simulink model "grid_traditional"  (R2023b)
settings: Solver=ode23s  StartTime=0.0  StopTime=32  RelTol=1e-3
values from neighbouring files (symbols this model uses):
  Ts = 5e-6    (= 5e-06)    [model_parameters.m]
undefined symbols (not defined in the file or in its folder): gcbh, Grid, IBR, L, SG, sps_rtmsupport, TX
libraries: spsThreePhaseVIMeasurementLib x13, spsFourierLib x13, spsPowerPositiveSequenceLib x13, spsThreePhaseSeriesRLCLoadLib x11, spsThreePhaseSeriesRLCBranchLib x10, spsThreePhaseTransformerTwoWindingsLib x10, spsDCVoltageSourceLib x8, spsFirstOrderFilterLib x8, spsabctodq0Lib x8, spsSimplifiedSynchronousMachinepuUnitsLib x6, spsGroundLib x4, spsUniversalBridgeLib x4
(part 1 of 2)
settings Model: SimulationMode=rapid-accelerator  Creator=psernatorre  LastModifiedBy=psernatorre
settings DataIOCC: InitialState=initial_data_trad2.xFinal  LoadInitialState=on  SaveFinalState=on  SaveOperatingPoint=on
settings GRTTargetCC: RTWCAPISignals=on  RTWCAPIParams=on

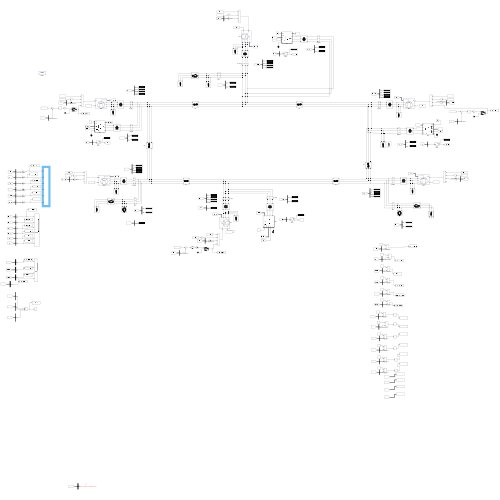
[thumbnail: Simulink's stored preview of the top-level diagram]
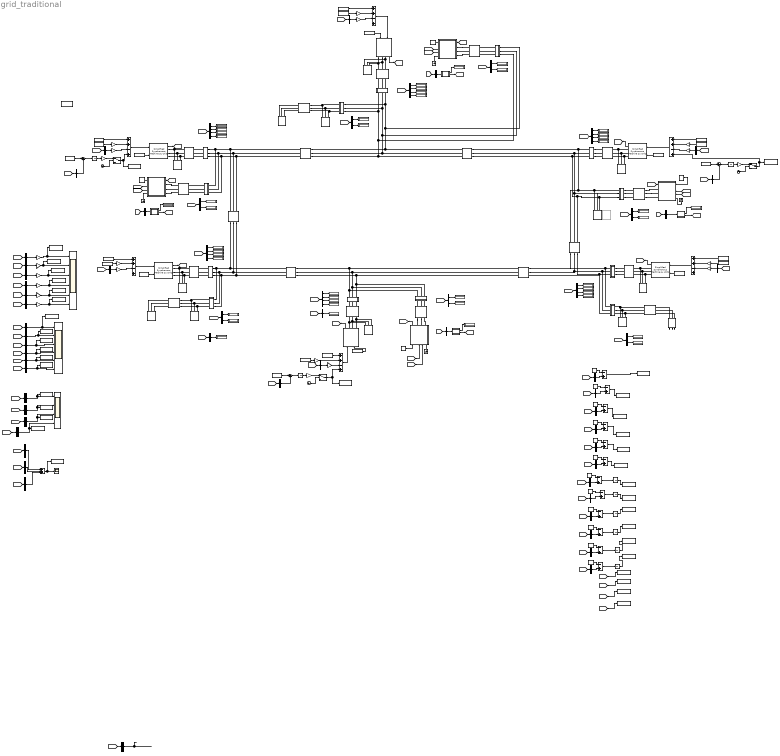
== system grid_traditional ==
  Add{,6..7,20..22} (6 alike) : Sum  Inputs=++-+
  Add1 : Sum  Inputs=+++
  Add{9,11..13,17..18,33..38} (12 alike) : Sum  Inputs=-+
  B1_IBR1 : Subsystem  mask{Sbase=Grid.Sbase, Vbase=Grid.Vbase, f=Grid.f, Ts=Ts, label=B1_IBR1, enable_power_calc=on}
      mask prompts: Sbase "Sbase (3-phase VA)"; Vbase "Vbase (L-L Vrms)"; f "Frequency (Hz)"; Ts "Sample time (s)"; label "Measure label"; enable_power_calc "Enable power calculation"
      mask init:
      | set_param([gcb '/signal'],'GotoTag', label)
      mask DialogControl DescGroupVar Prompt: Bus and measurements
      mask DialogControl Bus Prompt: Measure voltage, magnitude and phase, active power, reactive power
  B1_SG1 : Subsystem  mask{Sbase=Grid.Sbase, Vbase=Grid.Vbase, f=Grid.f, Ts=Ts, label=B1_SG1, enable_power_calc=on}
      mask prompts: Sbase "Sbase (3-phase VA)"; Vbase "Vbase (L-L Vrms)"; f "Frequency (Hz)"; Ts "Sample time (s)"; label "Measure label"; enable_power_calc "Enable power calculation"
      mask init:
      | set_param([gcb '/signal'],'GotoTag', label)
      mask DialogControl DescGroupVar Prompt: Bus and measurements
      mask DialogControl Bus Prompt: Measure voltage, magnitude and phase, active power, reactive power
  B5_L : Subsystem  mask{Sbase=Grid.Sbase, Vbase=Grid.Vbase, f=Grid.f, Ts=Ts, label=B5_L, enable_power_calc=on}
      mask prompts: Sbase "Sbase (3-phase VA)"; Vbase "Vbase (L-L Vrms)"; f "Frequency (Hz)"; Ts "Sample time (s)"; label "Measure label"; enable_power_calc "Enable power calculation"
      mask init:
      | set_param([gcb '/signal'],'GotoTag', label)
      mask DialogControl DescGroupVar Prompt: Bus and measurements
      mask DialogControl Bus Prompt: Measure voltage, magnitude and phase, active power, reactive power
  B5_SG6 : Subsystem  mask{Sbase=Grid.Sbase, Vbase=Grid.Vbase, f=Grid.f, Ts=Ts, label=B5_SG6, enable_power_calc=on}
      mask prompts: Sbase "Sbase (3-phase VA)"; Vbase "Vbase (L-L Vrms)"; f "Frequency (Hz)"; Ts "Sample time (s)"; label "Measure label"; enable_power_calc "Enable power calculation"
      mask init:
      | set_param([gcb '/signal'],'GotoTag', label)
      mask DialogControl DescGroupVar Prompt: Bus and measurements
      mask DialogControl Bus Prompt: Measure voltage, magnitude and phase, active power, reactive power
  B6_IBR3 : Subsystem  mask{Sbase=Grid.Sbase, Vbase=Grid.Vbase, f=Grid.f, Ts=Ts, label=B6_IBR3, enable_power_calc=on}
      mask prompts: Sbase "Sbase (3-phase VA)"; Vbase "Vbase (L-L Vrms)"; f "Frequency (Hz)"; Ts "Sample time (s)"; label "Measure label"; enable_power_calc "Enable power calculation"
      mask init:
      | set_param([gcb '/signal'],'GotoTag', label)
      mask DialogControl DescGroupVar Prompt: Bus and measurements
      mask DialogControl Bus Prompt: Measure voltage, magnitude and phase, active power, reactive power
  B6_SG5 : Subsystem  mask{Sbase=Grid.Sbase, Vbase=Grid.Vbase, f=Grid.f, Ts=Ts, label=B6_SG5, enable_power_calc=on}
      mask prompts: Sbase "Sbase (3-phase VA)"; Vbase "Vbase (L-L Vrms)"; f "Frequency (Hz)"; Ts "Sample time (s)"; label "Measure label"; enable_power_calc "Enable power calculation"
      mask init:
      | set_param([gcb '/signal'],'GotoTag', label)
      mask DialogControl DescGroupVar Prompt: Bus and measurements
      mask DialogControl Bus Prompt: Measure voltage, magnitude and phase, active power, reactive power
  B7_IBR4 : Subsystem  mask{Sbase=Grid.Sbase, Vbase=Grid.Vbase, f=Grid.f, Ts=Ts, label=B7_IBR4, enable_power_calc=on}
      mask prompts: Sbase "Sbase (3-phase VA)"; Vbase "Vbase (L-L Vrms)"; f "Frequency (Hz)"; Ts "Sample time (s)"; label "Measure label"; enable_power_calc "Enable power calculation"
      mask init:
      | set_param([gcb '/signal'],'GotoTag', label)
      mask DialogControl DescGroupVar Prompt: Bus and measurements
      mask DialogControl Bus Prompt: Measure voltage, magnitude and phase, active power, reactive power
  B7_L : Subsystem  mask{Sbase=Grid.Sbase, Vbase=Grid.Vbase, f=Grid.f, Ts=Ts, label=B7_L, enable_power_calc=on}
      mask prompts: Sbase "Sbase (3-phase VA)"; Vbase "Vbase (L-L Vrms)"; f "Frequency (Hz)"; Ts "Sample time (s)"; label "Measure label"; enable_power_calc "Enable power calculation"
      mask init:
      | set_param([gcb '/signal'],'GotoTag', label)
      mask DialogControl DescGroupVar Prompt: Bus and measurements
      mask DialogControl Bus Prompt: Measure voltage, magnitude and phase, active power, reactive power
  B7_SG4 : Subsystem  mask{Sbase=Grid.Sbase, Vbase=Grid.Vbase, f=Grid.f, Ts=Ts, label=B7_SG4, enable_power_calc=on}
      mask prompts: Sbase "Sbase (3-phase VA)"; Vbase "Vbase (L-L Vrms)"; f "Frequency (Hz)"; Ts "Sample time (s)"; label "Measure label"; enable_power_calc "Enable power calculation"
      mask init:
      | set_param([gcb '/signal'],'GotoTag', label)
      mask DialogControl DescGroupVar Prompt: Bus and measurements
      mask DialogControl Bus Prompt: Measure voltage, magnitude and phase, active power, reactive power
  B8_IBR2 : Subsystem  mask{Sbase=Grid.Sbase, Vbase=Grid.Vbase, f=Grid.f, Ts=Ts, label=B8_IBR2, enable_power_calc=on}
      mask prompts: Sbase "Sbase (3-phase VA)"; Vbase "Vbase (L-L Vrms)"; f "Frequency (Hz)"; Ts "Sample time (s)"; label "Measure label"; enable_power_calc "Enable power calculation"
      mask init:
      | set_param([gcb '/signal'],'GotoTag', label)
      mask DialogControl DescGroupVar Prompt: Bus and measurements
      mask DialogControl Bus Prompt: Measure voltage, magnitude and phase, active power, reactive power
  B8_SG3 : Subsystem  mask{Sbase=Grid.Sbase, Vbase=Grid.Vbase, f=Grid.f, Ts=Ts, label=B8_SG3, enable_power_calc=on}
      mask prompts: Sbase "Sbase (3-phase VA)"; Vbase "Vbase (L-L Vrms)"; f "Frequency (Hz)"; Ts "Sample time (s)"; label "Measure label"; enable_power_calc "Enable power calculation"
      mask init:
      | set_param([gcb '/signal'],'GotoTag', label)
      mask DialogControl DescGroupVar Prompt: Bus and measurements
      mask DialogControl Bus Prompt: Measure voltage, magnitude and phase, active power, reactive power
  B9_L : Subsystem  mask{Sbase=Grid.Sbase, Vbase=Grid.Vbase, f=Grid.f, Ts=Ts, label=B9_L, enable_power_calc=on}
      mask prompts: Sbase "Sbase (3-phase VA)"; Vbase "Vbase (L-L Vrms)"; f "Frequency (Hz)"; Ts "Sample time (s)"; label "Measure label"; enable_power_calc "Enable power calculation"
      mask init:
      | set_param([gcb '/signal'],'GotoTag', label)
      mask DialogControl DescGroupVar Prompt: Bus and measurements
      mask DialogControl Bus Prompt: Measure voltage, magnitude and phase, active power, reactive power
  B9_SG2 : Subsystem  mask{Sbase=Grid.Sbase, Vbase=Grid.Vbase, f=Grid.f, Ts=Ts, label=B9_SG2, enable_power_calc=on}
      mask prompts: Sbase "Sbase (3-phase VA)"; Vbase "Vbase (L-L Vrms)"; f "Frequency (Hz)"; Ts "Sample time (s)"; label "Measure label"; enable_power_calc "Enable power calculation"
      mask init:
      | set_param([gcb '/signal'],'GotoTag', label)
      mask DialogControl DescGroupVar Prompt: Bus and measurements
      mask DialogControl Bus Prompt: Measure voltage, magnitude and phase, active power, reactive power
  Bus Selector{1,29,31,33,91..92} (6 alike) : BusSelector  OutputSignals=P,Q,Vmag,Vphase
  Bus Selector{8,10..11,19,32,42..48,55,58} (14 alike) : BusSelector  OutputSignals=P
  Bus Selector{3..7,9,12..13,16..18,20..22,24..25,28,30,34,37,39..41,49..54} (29 alike) : BusSelector  OutputSignals=Rotor speed wm (pu)
  Bus Selector{14..15,35,56} (4 alike) : BusSelector  OutputSignals=V
  Bus Selector{2,23,26..27,36,38,57} (7 alike) : BusSelector  OutputSignals=P,Q
  Clock : Clock
  Clock1 : Clock
  Clock2 : Clock
  Constant{,17,20,23..24,28} (6 alike) : Constant  Value=1.02
  Constant1 : Constant  Value=0.54
  Constant{5..14,16,18..19,22,27,36..41} (21 alike) : Constant
  Constant15 : Constant  Value=0.52
  Constant2 : Constant  Value=0.35
  Constant21 : Constant  Value=0.10
  Constant25 : Constant  Value=0.80
  Constant26 : Constant  Value=0.70
  Constant29 : Constant  Value=0.15
  Constant3 : Constant  Value=0.35
  Constant30 : Constant  Value=0.30
  Constant4 : Constant  Value=0.35
  Display{1..44} (44 alike) : Display
      settings: Format=bank
  Gain{1,10..11,26..28} (6 alike) : Gain  Gain=Grid.f
  Gain12 : Gain  Gain=1/SG(4).Rp
  Gain17 : Gain  Gain=1/SG(2).Rp
  Gain18 : Gain  Gain=1/SG(2).Rp
  Gain19 : Gain  Gain=1/SG(3).Rp
  Gain2 : Gain  Gain=1/SG(1).Rp
  Gain20 : Gain  Gain=1/SG(3).Rp
  Gain21 : Gain  Gain=1/SG(4).Rp
  Gain22 : Gain  Gain=1/SG(5).Rp
  Gain23 : Gain  Gain=1/SG(5).Rp
  Gain24 : Gain  Gain=1/SG(6).Rp
  Gain25 : Gain  Gain=1/SG(6).Rp
  Gain3 : Gain  Gain=1/SG(1).Rp
  Gain4 : Gain  Gain=40
  Gain5 : Gain  Gain=40
  Gain6 : Gain  Gain=40
  Ground{1..4} (4 alike) : spsGroundLib/Ground  LConnTagsString=a
  IBR1 : Subsystem  mask{S=Grid.Sbase, V=IBR(1).Vbase, Vdc=IBR(1).Vdc, Rf=IBR(1).Rf, Lf=IBR(1).Lf, Rc=IBR(1).Rc, Lc=IBR(1).Lc, Kp=IBR(1).Kp, Ki=IBR(1).Ki, f=Grid.f, Tf=IBR(1).Tf, Ts=Ts, enable_state_estimation=off, A_est=0, B_est=0, C_est=0, D_est=0}
      mask prompts: S "Pnom (VA)"; V "Vnom (Line Vrms)"; Vdc "Vdc (V)"; Rf "Rf (p.u.)"; Lf "Lf (p.u.)"; Rc "Rc (p.u.)"; Lc "Lc (p.u.)"; f "Frequency (Hz)"; Tf "Tf (feed-forward)"; Ts "Sample time (s)"; enable_state_estimation "Enable state estimation"
      mask DialogControl DescGroupVar Prompt: PLL-based grid-following IBR with LC filter
      mask DialogControl DescTextVar Prompt: Implements a grid-following inverter with LC filter with PI controllers in dq0-synchronous frames. It considers feed-forward compensation with first-order low-pass filter. Rf and Lf are impendances of the internal filter, and Rc and Lc are the impendances including a step-up transformer if there exists.
      mask Display: image('GFL_LC.png');
  IBR2 : Subsystem  mask{S=Grid.Sbase, V=IBR(2).Vbase, Vdc=IBR(2).Vdc, Rf=IBR(2).Rf, Lf=IBR(2).Lf, Rc=IBR(2).Rc, Lc=IBR(2).Lc, Kp=IBR(2).Kp, Ki=IBR(2).Ki, f=Grid.f, Tf=IBR(2).Tf, Ts=Ts, enable_state_estimation=off, A_est=0, B_est=0, C_est=0, D_est=0}
      mask prompts: S "Pnom (VA)"; V "Vnom (Line Vrms)"; Vdc "Vdc (V)"; Rf "Rf (p.u.)"; Lf "Lf (p.u.)"; Rc "Rc (p.u.)"; Lc "Lc (p.u.)"; f "Frequency (Hz)"; Tf "Tf (feed-forward)"; Ts "Sample time (s)"; enable_state_estimation "Enable state estimation"
      mask DialogControl DescGroupVar Prompt: PLL-based grid-following IBR with LC filter
      mask DialogControl DescTextVar Prompt: Implements a grid-following inverter with LC filter with PI controllers in dq0-synchronous frames. It considers feed-forward compensation with first-order low-pass filter. Rf and Lf are impendances of the internal filter, and Rc and Lc are the impendances including a step-up transformer if there exists.
      mask Display: image('GFL_LC.png');
  IBR3 : Subsystem  mask{S=Grid.Sbase, V=IBR(3).Vbase, Vdc=IBR(3).Vdc, Rf=IBR(3).Rf, Lf=IBR(3).Lf, Rc=IBR(3).Rc, Lc=IBR(3).Lc, Kp=IBR(3).Kp, Ki=IBR(3).Ki, f=Grid.f, Tf=IBR(3).Tf, Ts=Ts, enable_state_estimation=off, A_est=0, B_est=0, C_est=0, D_est=0}
      mask prompts: S "Pnom (VA)"; V "Vnom (Line Vrms)"; Vdc "Vdc (V)"; Rf "Rf (p.u.)"; Lf "Lf (p.u.)"; Rc "Rc (p.u.)"; Lc "Lc (p.u.)"; f "Frequency (Hz)"; Tf "Tf (feed-forward)"; Ts "Sample time (s)"; enable_state_estimation "Enable state estimation"
      mask DialogControl DescGroupVar Prompt: PLL-based grid-following IBR with LC filter
      mask DialogControl DescTextVar Prompt: Implements a grid-following inverter with LC filter with PI controllers in dq0-synchronous frames. It considers feed-forward compensation with first-order low-pass filter. Rf and Lf are impendances of the internal filter, and Rc and Lc are the impendances including a step-up transformer if there exists.
      mask Display: image('GFL_LC.png');
  IBR4 : Subsystem  mask{S=Grid.Sbase, V=IBR(2).Vbase, Vdc=IBR(2).Vdc, Rf=IBR(2).Rf, Lf=IBR(2).Lf, Rc=IBR(2).Rc, Lc=IBR(2).Lc, Kp=IBR(2).Kp, Ki=IBR(2).Ki, f=Grid.f, Tf=IBR(2).Tf, Ts=Ts, enable_state_estimation=off, A_est=0, B_est=0, C_est=0, D_est=0}
      mask prompts: S "Pnom (VA)"; V "Vnom (Line Vrms)"; Vdc "Vdc (V)"; Rf "Rf (p.u.)"; Lf "Lf (p.u.)"; Rc "Rc (p.u.)"; Lc "Lc (p.u.)"; f "Frequency (Hz)"; Tf "Tf (feed-forward)"; Ts "Sample time (s)"; enable_state_estimation "Enable state estimation"
      mask DialogControl DescGroupVar Prompt: PLL-based grid-following IBR with LC filter
      mask DialogControl DescTextVar Prompt: Implements a grid-following inverter with LC filter with PI controllers in dq0-synchronous frames. It considers feed-forward compensation with first-order low-pass filter. Rf and Lf are impendances of the internal filter, and Rc and Lc are the impendances including a step-up transformer if there exists.
      mask Display: image('GFL_LC.png');
  Integrator{,1..5,12..14} (9 alike) : Integrator
  PLL (3ph) : Subsystem  AncestorBlock=|  DialogController=POWERSYS.PowerSysDialog  LoadFcn=sps_rtmsupport('LoadFcn', gcbh);  StartFcn=sps_rtmsupport('StartFcn', gcbh);  StopFcn=sps_rtmsupport('StopFcn', gcbh);  mask(PLL (3ph)){Fmin=45, Par_Init=[0, 60], ParK=[180, 3200, 1], TcD=1e-4, MaxRateChangeFreq=12, FilterCutOffFreq=25, Ts=Ts, AGC=on}
      | sps_lib/Control/PLL
      | (3ph)
      mask prompts: Fmin "Minimum frequency (Hz):"; Par_Init "Initial inputs [ Phase (degrees), Frequency (Hz) ]:"; ParK "Regulator gains [ Kp, Ki, Kd ]:"; TcD "Time constant for derivative action (s):"; MaxRateChangeFreq "Maximum rate of change of frequency (Hz/s):"; FilterCutOffFreq "Filter cut-off frequency for frequency measurement (Hz):"; Ts "Sample time:"; AGC "Enable automatic gain control"
      mask help:
      | This Phase Locked Loop (PLL) system can be used  to synchronize on a set of variable frequency, three-phase sinusoidal signals. If the Automatic Gain Control is enabled, the input (phase error) of the PLL regulator is scaled according to the input signals magnitude.
      |
      | For optimal performance, set regulator gains [ Kp Ki  Kd ] = [ 180  3200  1 ] and check the Enable Automatic Gain Control parameter.
      |
      | Input : Vector containing the normalized three-phase signals [Va Vb Vc]
      | Output 1:  Measured frequency (Hz) = w/(2pi)
      | Output 2:  Ramp w.t varying between  0 and 2*pi, synchronized on zero crossings of the fundamental (positive-sequence) of phase A.
      mask init:
      | block=gcb;
      | [WantBlockChoice,Ts,sps] = powericon('PLL3phInit',block,Fmin,Par_Init,ParK,TcD, MaxRateChangeFreq, FilterCutOffFreq, AGC,Ts);
      | powericon('SetInternalModels','set',block,WantBlockChoice);
      settings: CopyFcn=sps_rtmsupport('CopyFcn', gcbh);  DeleteFcn=sps_rtmsupport('DeleteFcn', gcbh);  UndoDeleteFcn=sps_rtmsupport('UndoDeleteFcn', gcbh);  ModelCloseFcn=sps_rtmsupport('ModelCloseFcn', gcbh);  PreSaveFcn=sps_rtmsupport('PreSaveFcn', gcbh);  PostSaveFcn=sps_rtmsupport('PostSaveFcn', gcbh);  NameChangeFcn=sps_rtmsupport('NameChangeFcn', gcbh);  PreCopyFcn=sps_rtmsupport('PreCopyFcn', gcbh);  OpenFcn=sps_rtmsupport('OpenFcn', gcbh, [8]);  CloseFcn=sps_rtmsupport('CloseFcn', gcbh);  PreDeleteFcn=sps_rtmsupport('PreDeleteFcn', gcbh);
      settings: LibrarySourceBlock=|
      | sps_lib/Control/PLL
      | (3ph)
      mask Help: helpview(psbhelp);
  PLL (3ph)1 : Subsystem  AncestorBlock=|  DialogController=POWERSYS.PowerSysDialog  LoadFcn=sps_rtmsupport('LoadFcn', gcbh);  StartFcn=sps_rtmsupport('StartFcn', gcbh);  StopFcn=sps_rtmsupport('StopFcn', gcbh);  mask(PLL (3ph)){Fmin=45, Par_Init=[0, 60], ParK=[180, 3200, 1], TcD=1e-4, MaxRateChangeFreq=12, FilterCutOffFreq=25, Ts=Ts, AGC=on}
      | sps_lib/Control/PLL
      | (3ph)
      mask prompts: Fmin "Minimum frequency (Hz):"; Par_Init "Initial inputs [ Phase (degrees), Frequency (Hz) ]:"; ParK "Regulator gains [ Kp, Ki, Kd ]:"; TcD "Time constant for derivative action (s):"; MaxRateChangeFreq "Maximum rate of change of frequency (Hz/s):"; FilterCutOffFreq "Filter cut-off frequency for frequency measurement (Hz):"; Ts "Sample time:"; AGC "Enable automatic gain control"
      mask help:
      | This Phase Locked Loop (PLL) system can be used  to synchronize on a set of variable frequency, three-phase sinusoidal signals. If the Automatic Gain Control is enabled, the input (phase error) of the PLL regulator is scaled according to the input signals magnitude.
      |
      | For optimal performance, set regulator gains [ Kp Ki  Kd ] = [ 180  3200  1 ] and check the Enable Automatic Gain Control parameter.
      |
      | Input : Vector containing the normalized three-phase signals [Va Vb Vc]
      | Output 1:  Measured frequency (Hz) = w/(2pi)
      | Output 2:  Ramp w.t varying between  0 and 2*pi, synchronized on zero crossings of the fundamental (positive-sequence) of phase A.
      mask init:
      | block=gcb;
      | [WantBlockChoice,Ts,sps] = powericon('PLL3phInit',block,Fmin,Par_Init,ParK,TcD, MaxRateChangeFreq, FilterCutOffFreq, AGC,Ts);
      | powericon('SetInternalModels','set',block,WantBlockChoice);
      settings: CopyFcn=sps_rtmsupport('CopyFcn', gcbh);  DeleteFcn=sps_rtmsupport('DeleteFcn', gcbh);  UndoDeleteFcn=sps_rtmsupport('UndoDeleteFcn', gcbh);  ModelCloseFcn=sps_rtmsupport('ModelCloseFcn', gcbh);  PreSaveFcn=sps_rtmsupport('PreSaveFcn', gcbh);  PostSaveFcn=sps_rtmsupport('PostSaveFcn', gcbh);  NameChangeFcn=sps_rtmsupport('NameChangeFcn', gcbh);  PreCopyFcn=sps_rtmsupport('PreCopyFcn', gcbh);  OpenFcn=sps_rtmsupport('OpenFcn', gcbh, [8]);  CloseFcn=sps_rtmsupport('CloseFcn', gcbh);  PreDeleteFcn=sps_rtmsupport('PreDeleteFcn', gcbh);
      settings: LibrarySourceBlock=|
      | sps_lib/Control/PLL
      | (3ph)
      mask Help: helpview(psbhelp);
  PLL (3ph)2 : Subsystem  AncestorBlock=|  DialogController=POWERSYS.PowerSysDialog  LoadFcn=sps_rtmsupport('LoadFcn', gcbh);  StartFcn=sps_rtmsupport('StartFcn', gcbh);  StopFcn=sps_rtmsupport('StopFcn', gcbh);  mask(PLL (3ph)){Fmin=45, Par_Init=[0, 60], ParK=[180, 3200, 1], TcD=1e-4, MaxRateChangeFreq=12, FilterCutOffFreq=25, Ts=Ts, AGC=on}
      | sps_lib/Control/PLL
      | (3ph)
      mask prompts: Fmin "Minimum frequency (Hz):"; Par_Init "Initial inputs [ Phase (degrees), Frequency (Hz) ]:"; ParK "Regulator gains [ Kp, Ki, Kd ]:"; TcD "Time constant for derivative action (s):"; MaxRateChangeFreq "Maximum rate of change of frequency (Hz/s):"; FilterCutOffFreq "Filter cut-off frequency for frequency measurement (Hz):"; Ts "Sample time:"; AGC "Enable automatic gain control"
      mask help:
      | This Phase Locked Loop (PLL) system can be used  to synchronize on a set of variable frequency, three-phase sinusoidal signals. If the Automatic Gain Control is enabled, the input (phase error) of the PLL regulator is scaled according to the input signals magnitude.
      |
      | For optimal performance, set regulator gains [ Kp Ki  Kd ] = [ 180  3200  1 ] and check the Enable Automatic Gain Control parameter.
      |
      | Input : Vector containing the normalized three-phase signals [Va Vb Vc]
      | Output 1:  Measured frequency (Hz) = w/(2pi)
      | Output 2:  Ramp w.t varying between  0 and 2*pi, synchronized on zero crossings of the fundamental (positive-sequence) of phase A.
      mask init:
      | block=gcb;
      | [WantBlockChoice,Ts,sps] = powericon('PLL3phInit',block,Fmin,Par_Init,ParK,TcD, MaxRateChangeFreq, FilterCutOffFreq, AGC,Ts);
      | powericon('SetInternalModels','set',block,WantBlockChoice);
      settings: CopyFcn=sps_rtmsupport('CopyFcn', gcbh);  DeleteFcn=sps_rtmsupport('DeleteFcn', gcbh);  UndoDeleteFcn=sps_rtmsupport('UndoDeleteFcn', gcbh);  ModelCloseFcn=sps_rtmsupport('ModelCloseFcn', gcbh);  PreSaveFcn=sps_rtmsupport('PreSaveFcn', gcbh);  PostSaveFcn=sps_rtmsupport('PostSaveFcn', gcbh);  NameChangeFcn=sps_rtmsupport('NameChangeFcn', gcbh);  PreCopyFcn=sps_rtmsupport('PreCopyFcn', gcbh);  OpenFcn=sps_rtmsupport('OpenFcn', gcbh, [8]);  CloseFcn=sps_rtmsupport('CloseFcn', gcbh);  PreDeleteFcn=sps_rtmsupport('PreDeleteFcn', gcbh);
      settings: LibrarySourceBlock=|
      | sps_lib/Control/PLL
      | (3ph)
      mask Help: helpview(psbhelp);
  PLL (3ph)3 : Subsystem  AncestorBlock=|  DialogController=POWERSYS.PowerSysDialog  LoadFcn=sps_rtmsupport('LoadFcn', gcbh);  StartFcn=sps_rtmsupport('StartFcn', gcbh);  StopFcn=sps_rtmsupport('StopFcn', gcbh);  mask(PLL (3ph)){Fmin=45, Par_Init=[0, 60], ParK=[180, 3200, 1], TcD=1e-4, MaxRateChangeFreq=12, FilterCutOffFreq=25, Ts=Ts, AGC=on}
      | sps_lib/Control/PLL
      | (3ph)
      mask prompts: Fmin "Minimum frequency (Hz):"; Par_Init "Initial inputs [ Phase (degrees), Frequency (Hz) ]:"; ParK "Regulator gains [ Kp, Ki, Kd ]:"; TcD "Time constant for derivative action (s):"; MaxRateChangeFreq "Maximum rate of change of frequency (Hz/s):"; FilterCutOffFreq "Filter cut-off frequency for frequency measurement (Hz):"; Ts "Sample time:"; AGC "Enable automatic gain control"
      mask help:
      | This Phase Locked Loop (PLL) system can be used  to synchronize on a set of variable frequency, three-phase sinusoidal signals. If the Automatic Gain Control is enabled, the input (phase error) of the PLL regulator is scaled according to the input signals magnitude.
      |
      | For optimal performance, set regulator gains [ Kp Ki  Kd ] = [ 180  3200  1 ] and check the Enable Automatic Gain Control parameter.
      |
      | Input : Vector containing the normalized three-phase signals [Va Vb Vc]
      | Output 1:  Measured frequency (Hz) = w/(2pi)
      | Output 2:  Ramp w.t varying between  0 and 2*pi, synchronized on zero crossings of the fundamental (positive-sequence) of phase A.
      mask init:
      | block=gcb;
      | [WantBlockChoice,Ts,sps] = powericon('PLL3phInit',block,Fmin,Par_Init,ParK,TcD, MaxRateChangeFreq, FilterCutOffFreq, AGC,Ts);
      | powericon('SetInternalModels','set',block,WantBlockChoice);
      settings: CopyFcn=sps_rtmsupport('CopyFcn', gcbh);  DeleteFcn=sps_rtmsupport('DeleteFcn', gcbh);  UndoDeleteFcn=sps_rtmsupport('UndoDeleteFcn', gcbh);  ModelCloseFcn=sps_rtmsupport('ModelCloseFcn', gcbh);  PreSaveFcn=sps_rtmsupport('PreSaveFcn', gcbh);  PostSaveFcn=sps_rtmsupport('PostSaveFcn', gcbh);  NameChangeFcn=sps_rtmsupport('NameChangeFcn', gcbh);  PreCopyFcn=sps_rtmsupport('PreCopyFcn', gcbh);  OpenFcn=sps_rtmsupport('OpenFcn', gcbh, [8]);  CloseFcn=sps_rtmsupport('CloseFcn', gcbh);  PreDeleteFcn=sps_rtmsupport('PreDeleteFcn', gcbh);
      settings: LibrarySourceBlock=|
      | sps_lib/Control/PLL
      | (3ph)
      mask Help: helpview(psbhelp);
  SG1 : spsSimplifiedSynchronousMachinepuUnitsLib/Simplified Synchronous Machine pu Units  ConnectionType=3-wire Y  MechanicalLoad=Mechanical power Pm  MeasurementBus=off  NominalParameters=[SG(1).Sbase SG(1).Vbase Grid.f]  Mechanical=[SG(1).H SG(1).KD 20]  InternalRL="[0.02  0.3]"  InitialConditions=[0 6.93594 0.40802 0.40802 0.40802 0.604989 -119.395 120.605]  IterativeDiscreteModel=Trapezoidal non iterative  TsBlock=-1  TsPowergui=0  LoadFlowParameters=[1,0,0,0,0]  Units=0  BusType=swing  Pref=20000000  Qref=0  Qmin=-Inf  Qmax=Inf  PLF=0  QLF=0
      settings: LibrarySourceBlock=|
      | sps_lib/Electrical Machines/Simplified Synchronous
      | Machine pu Units
  SG2 : spsSimplifiedSynchronousMachinepuUnitsLib/Simplified Synchronous Machine pu Units  ConnectionType=3-wire Y  MechanicalLoad=Mechanical power Pm  MeasurementBus=off  NominalParameters=[SG(2).Sbase SG(2).Vbase Grid.f]  Mechanical=[SG(2).H SG(2).KD 20]  InternalRL="[0.02  0.3]"  InitialConditions=[0 1.16591 0.202284 0.202284 0.202284 -10.8065 -130.807 109.193]  IterativeDiscreteModel=Trapezoidal non iterative  TsBlock=-1  TsPowergui=0  LoadFlowParameters=[1,0,0,0,0]  Units=0  BusType=PV  Pref=20000000  Qref=0  Qmin=-Inf  Qmax=Inf  PLF=0  QLF=0
      settings: LibrarySourceBlock=|
      | sps_lib/Electrical Machines/Simplified Synchronous
      | Machine pu Units
  SG3 : spsSimplifiedSynchronousMachinepuUnitsLib/Simplified Synchronous Machine pu Units  ConnectionType=3-wire Y  MechanicalLoad=Mechanical power Pm  MeasurementBus=off  NominalParameters=[SG(3).Sbase SG(3).Vbase Grid.f]  Mechanical=[SG(3).H SG(3).KD 20]  InternalRL="[0.02  0.3]"  InitialConditions=[0 2.15966 0.200038 0.200038 0.200038 -0.157653 -120.158 119.842]  IterativeDiscreteModel=Trapezoidal non iterative  TsBlock=-1  TsPowergui=0  LoadFlowParameters=[1,0,0,0,0]  Units=0  BusType=PV  Pref=20000000  Qref=0  Qmin=-Inf  Qmax=Inf  PLF=0  QLF=0
      settings: LibrarySourceBlock=|
      | sps_lib/Electrical Machines/Simplified Synchronous
      | Machine pu Units
  SG4 : spsSimplifiedSynchronousMachinepuUnitsLib/Simplified Synchronous Machine pu Units  ConnectionType=3-wire Y  MechanicalLoad=Mechanical power Pm  MeasurementBus=off  NominalParameters=[SG(4).Sbase SG(4).Vbase Grid.f]  Mechanical=[SG(4).H SG(4).KD 20]  InternalRL="[0.02  0.3]"  InitialConditions=[0 -3.45004 0.102056 0.102056 0.102056 -16.653 -136.653 103.347]  IterativeDiscreteModel=Trapezoidal non iterative  TsBlock=-1  TsPowergui=0  LoadFlowParameters=[1,0,0,0,0]  Units=0  BusType=PV  Pref=10000000  Qref=0  Qmin=-Inf  Qmax=Inf  PLF=0  QLF=0
      settings: LibrarySourceBlock=|
      | sps_lib/Electrical Machines/Simplified Synchronous
      | Machine pu Units
  SG5 : spsSimplifiedSynchronousMachinepuUnitsLib/Simplified Synchronous Machine pu Units  ConnectionType=3-wire Y  MechanicalLoad=Mechanical power Pm  MeasurementBus=off  NominalParameters=[SG(5).Sbase SG(5).Vbase Grid.f]  Mechanical=[SG(5).H SG(5).KD 20]  InternalRL="[0.02  0.3]"  InitialConditions=[0 -3.45004 0.102056 0.102056 0.102056 -16.653 -136.653 103.347]  IterativeDiscreteModel=Trapezoidal non iterative  TsBlock=-1  TsPowergui=0  LoadFlowParameters=[1,0,0,0,0]  Units=0  BusType=PV  Pref=10000000  Qref=0  Qmin=-Inf  Qmax=Inf  PLF=0  QLF=0
      settings: LibrarySourceBlock=|
      | sps_lib/Electrical Machines/Simplified Synchronous
      | Machine pu Units
  SG6 : spsSimplifiedSynchronousMachinepuUnitsLib/Simplified Synchronous Machine pu Units  ConnectionType=3-wire Y  MechanicalLoad=Mechanical power Pm  MeasurementBus=off  NominalParameters=[SG(6).Sbase SG(6).Vbase Grid.f]  Mechanical=[SG(6).H SG(6).KD 20]  InternalRL="[0.02  0.3]"  InitialConditions=[0 -3.45004 0.102056 0.102056 0.102056 -16.653 -136.653 103.347]  IterativeDiscreteModel=Trapezoidal non iterative  TsBlock=-1  TsPowergui=0  LoadFlowParameters=[1,0,0,0,0]  Units=0  BusType=PV  Pref=10000000  Qref=0  Qmin=-Inf  Qmax=Inf  PLF=0  QLF=0
      settings: LibrarySourceBlock=|
      | sps_lib/Electrical Machines/Simplified Synchronous
      | Machine pu Units
  Scope : Scope  NumInputPorts=6
  Scope1 : Scope  NumInputPorts=6
  Scope2 : Scope  NumInputPorts=4
  Scope3 : Scope
  Sum : Sum  Inputs=|+-
  Sum1 : Sum  Inputs=|+-
  Sum2 : Sum  Inputs=|+-
  Switch : Switch  Threshold=3  SaturateOnIntegerOverflow=off  InputSameDT=off
  Switch1 : Switch  Threshold=3  SaturateOnIntegerOverflow=off  InputSameDT=off
  Switch2 : Switch  Threshold=3  SaturateOnIntegerOverflow=off  InputSameDT=off
  TX1 : spsThreePhaseSeriesRLCBranchLib/Three-Phase Series RLC Branch  LConnTagsString=A|B|C  RConnTagsString=A|B|C  BranchType=RL  Resistance=TX(1).R_ohm  Inductance=TX(1).L_H  Capacitance=1e-6  Measurements=None
  TX2 : spsThreePhaseSeriesRLCBranchLib/Three-Phase Series RLC Branch  LConnTagsString=A|B|C  RConnTagsString=A|B|C  BranchType=RL  Resistance=TX(2).R_ohm  Inductance=TX(2).L_H  Capacitance=1e-6  Measurements=None
  TX3 : spsThreePhaseSeriesRLCBranchLib/Three-Phase Series RLC Branch  LConnTagsString=A|B|C  RConnTagsString=A|B|C  BranchType=RL  Resistance=TX(3).R_ohm  Inductance=TX(3).L_H  Capacitance=1e-6  Measurements=None
  TX4 : spsThreePhaseSeriesRLCBranchLib/Three-Phase Series RLC Branch  LConnTagsString=A|B|C  RConnTagsString=A|B|C  BranchType=RL  Resistance=TX(4).R_ohm  Inductance=TX(4).L_H  Capacitance=1e-6  Measurements=None
  TX5 : spsThreePhaseSeriesRLCBranchLib/Three-Phase Series RLC Branch  LConnTagsString=A|B|C  RConnTagsString=A|B|C  BranchType=RL  Resistance=TX(5).R_ohm  Inductance=TX(5).L_H  Capacitance=1e-6  Measurements=None
  TX6 : spsThreePhaseSeriesRLCBranchLib/Three-Phase Series RLC Branch  LConnTagsString=A|B|C  RConnTagsString=A|B|C  BranchType=RL  Resistance=TX(6).R_ohm  Inductance=TX(6).L_H  Capacitance=1e-6  Measurements=None
  Three-Phase Parallel RLC Load : spsThreePhaseParallelRLCLoadLib/Three-Phase Parallel RLC Load  LConnTagsString=A|B|C  Configuration=Y (grounded)  NominalVoltage=Grid.Vbase  Vabc=[1e3 1e3 1e3]  Vabcp=[1e3 1e3 1e3]  NominalFrequency=60  UnbalancedPower=off  ActivePower=L(5).P  InductivePower=0  CapacitivePower=L(5).QC  Pabc=[10e3 9e3 11e3]  QLabc=[100 90 110]  QCabc=[100 90 110]  Pabcp=[10e3 9e3 11e3]  QLabcp=[100 90 110]  QCabcp=[100 90 110]  Measurements=None  LoadType=constant Z
  Three-Phase Parallel RLC Load1 : spsThreePhaseParallelRLCLoadLib/Three-Phase Parallel RLC Load  LConnTagsString=A|B|C  Configuration=Y (grounded)  NominalVoltage=(229163)*1.00253  Vabc=[1e3 1e3 1e3]  Vabcp=[1e3 1e3 1e3]  NominalFrequency=60  UnbalancedPower=off  ActivePower=20000000  InductivePower=0  CapacitivePower=0  Pabc=[10e3 9e3 11e3]  QLabc=[100 90 110]  QCabc=[100 90 110]  Pabcp=[10e3 9e3 11e3]  QLabcp=[100 90 110]  QCabcp=[100 90 110]  Measurements=None  LoadType=constant Z
  Three-Phase Parallel RLC Load2 : spsThreePhaseParallelRLCLoadLib/Three-Phase Parallel RLC Load  LConnTagsString=A|B|C  Configuration=Y (grounded)  NominalVoltage=Grid.Vbase  Vabc=[1e3 1e3 1e3]  Vabcp=[1e3 1e3 1e3]  NominalFrequency=60  UnbalancedPower=off  ActivePower=L(1).P  InductivePower=0  CapacitivePower=L(1).QC  Pabc=[10e3 9e3 11e3]  QLabc=[100 90 110]  QCabc=[100 90 110]  Pabcp=[10e3 9e3 11e3]  QLabcp=[100 90 110]  QCabcp=[100 90 110]  Measurements=None  LoadType=constant Z
  Three-Phase Series RLC Load1 : spsThreePhaseSeriesRLCLoadLib/Three-Phase Series RLC Load  LConnTagsString=A|B|C  Configuration=Y (grounded)  NominalVoltage=Grid.Vbase  Vabc=[1e3 1e3 1e3]  Vabcp=[1e3 1e3 1e3]  NominalFrequency=Grid.f  UnbalancedPower=off  ActivePower=L(2).P*1  InductivePower=0  CapacitivePower=0  Pabc=[10e3 9e3 11e3]  QLabc=[100 90 110]  QCabc=[100 90 110]  Pabcp=[10e3 9e3 11e3]  QLabcp=[100 90 110]  QCabcp=[100 90 110]  Measurements=None  LoadType=constant Z
  Three-Phase Series RLC Load10 : spsThreePhaseSeriesRLCLoadLib/Three-Phase Series RLC Load  LConnTagsString=A|B|C  Configuration=Y (grounded)  NominalVoltage=Grid.Vbase  Vabc=[1e3 1e3 1e3]  Vabcp=[1e3 1e3 1e3]  NominalFrequency=Grid.f  UnbalancedPower=off  ActivePower=L(6).P  InductivePower=0  CapacitivePower=0  Pabc=[10e3 9e3 11e3]  QLabc=[100 90 110]  QCabc=[100 90 110]  Pabcp=[10e3 9e3 11e3]  QLabcp=[100 90 110]  QCabcp=[100 90 110]  Measurements=None  LoadType=constant Z
  Three-Phase Series RLC Load11 : spsThreePhaseSeriesRLCLoadLib/Three-Phase Series RLC Load  LConnTagsString=A|B|C  Configuration=Y (grounded)  NominalVoltage=SG(2).Vbase  Vabc=[1e3 1e3 1e3]  Vabcp=[1e3 1e3 1e3]  NominalFrequency=Grid.f  UnbalancedPower=off  ActivePower=10000000  InductivePower=0  CapacitivePower=0  Pabc=[10e3 9e3 11e3]  QLabc=[100 90 110]  QCabc=[100 90 110]  Pabcp=[10e3 9e3 11e3]  QLabcp=[100 90 110]  QCabcp=[100 90 110]  Measurements=None  LoadType=constant Z
  Three-Phase Series RLC Load13 : spsThreePhaseSeriesRLCLoadLib/Three-Phase Series RLC Load  Commented=on  LConnTagsString=A|B|C  Configuration=Y (grounded)  NominalVoltage=(229163)*1.00253  Vabc=[1e3 1e3 1e3]  Vabcp=[1e3 1e3 1e3]  NominalFrequency=Grid.f  UnbalancedPower=off  ActivePower=20000000  InductivePower=0  CapacitivePower=0  Pabc=[10e3 9e3 11e3]  QLabc=[100 90 110]  QCabc=[100 90 110]  Pabcp=[10e3 9e3 11e3]  QLabcp=[100 90 110]  QCabcp=[100 90 110]  Measurements=None  LoadType=constant Z
  Three-Phase Series RLC Load2 : spsThreePhaseSeriesRLCLoadLib/Three-Phase Series RLC Load  LConnTagsString=A|B|C  Configuration=Y (grounded)  NominalVoltage=SG(1).Vbase  Vabc=[1e3 1e3 1e3]  Vabcp=[1e3 1e3 1e3]  NominalFrequency=Grid.f  UnbalancedPower=off  ActivePower=20000000  InductivePower=0  CapacitivePower=0  Pabc=[10e3 9e3 11e3]  QLabc=[100 90 110]  QCabc=[100 90 110]  Pabcp=[10e3 9e3 11e3]  QLabcp=[100 90 110]  QCabcp=[100 90 110]  Measurements=None  LoadType=constant Z
  Three-Phase Series RLC Load3 : spsThreePhaseSeriesRLCLoadLib/Three-Phase Series RLC Load  LConnTagsString=A|B|C  Configuration=Y (grounded)  NominalVoltage=(229163)*1.00253  Vabc=[1e3 1e3 1e3]  Vabcp=[1e3 1e3 1e3]  NominalFrequency=Grid.f  UnbalancedPower=off  ActivePower=L(3).P  InductivePower=0  CapacitivePower=0  Pabc=[10e3 9e3 11e3]  QLabc=[100 90 110]  QCabc=[100 90 110]  Pabcp=[10e3 9e3 11e3]  QLabcp=[100 90 110]  QCabcp=[100 90 110]  Measurements=None  LoadType=constant PQ
  Three-Phase Series RLC Load4 : spsThreePhaseSeriesRLCLoadLib/Three-Phase Series RLC Load  LConnTagsString=A|B|C  Configuration=Y (grounded)  NominalVoltage=SG(2).Vbase  Vabc=[1e3 1e3 1e3]  Vabcp=[1e3 1e3 1e3]  NominalFrequency=Grid.f  UnbalancedPower=off  ActivePower=5000000  InductivePower=0  CapacitivePower=0  Pabc=[10e3 9e3 11e3]  QLabc=[100 90 110]  QCabc=[100 90 110]  Pabcp=[10e3 9e3 11e3]  QLabcp=[100 90 110]  QCabcp=[100 90 110]  Measurements=None  LoadType=constant Z
  Three-Phase Series RLC Load5 : spsThreePhaseSeriesRLCLoadLib/Three-Phase Series RLC Load  LConnTagsString=A|B|C  Configuration=Y (grounded)  NominalVoltage=SG(2).Vbase  Vabc=[1e3 1e3 1e3]  Vabcp=[1e3 1e3 1e3]  NominalFrequency=Grid.f  UnbalancedPower=off  ActivePower=10000000  InductivePower=0  CapacitivePower=0  Pabc=[10e3 9e3 11e3]  QLabc=[100 90 110]  QCabc=[100 90 110]  Pabcp=[10e3 9e3 11e3]  QLabcp=[100 90 110]  QCabcp=[100 90 110]  Measurements=None  LoadType=constant Z
  Three-Phase Series RLC Load6 : spsThreePhaseSeriesRLCLoadLib/Three-Phase Series RLC Load  LConnTagsString=A|B|C  Configuration=Y (grounded)  NominalVoltage=Grid.Vbase  Vabc=[1e3 1e3 1e3]  Vabcp=[1e3 1e3 1e3]  NominalFrequency=Grid.f  UnbalancedPower=off  ActivePower=L(2).P*2  InductivePower=0  CapacitivePower=0  Pabc=[10e3 9e3 11e3]  QLabc=[100 90 110]  QCabc=[100 90 110]  Pabcp=[10e3 9e3 11e3]  QLabcp=[100 90 110]  QCabcp=[100 90 110]  Measurements=None  LoadType=constant Z
  Three-Phase Series RLC Load7 : spsThreePhaseSeriesRLCLoadLib/Three-Phase Series RLC Load  LConnTagsString=A|B|C  Configuration=Y (grounded)  NominalVoltage=SG(2).Vbase  Vabc=[1e3 1e3 1e3]  Vabcp=[1e3 1e3 1e3]  NominalFrequency=Grid.f  UnbalancedPower=off  ActivePower=10000000  InductivePower=0  CapacitivePower=0  Pabc=[10e3 9e3 11e3]  QLabc=[100 90 110]  QCabc=[100 90 110]  Pabcp=[10e3 9e3 11e3]  QLabcp=[100 90 110]  QCabcp=[100 90 110]  Measurements=None  LoadType=constant Z
  Three-Phase Series RLC Load8 : spsThreePhaseSeriesRLCLoadLib/Three-Phase Series RLC Load  LConnTagsString=A|B|C  Configuration=Y (grounded)  NominalVoltage=SG(2).Vbase  Vabc=[1e3 1e3 1e3]  Vabcp=[1e3 1e3 1e3]  NominalFrequency=Grid.f  UnbalancedPower=off  ActivePower=5000000  InductivePower=0  CapacitivePower=0  Pabc=[10e3 9e3 11e3]  QLabc=[100 90 110]  QCabc=[100 90 110]  Pabcp=[10e3 9e3 11e3]  QLabcp=[100 90 110]  QCabcp=[100 90 110]  Measurements=None  LoadType=constant Z
  Three-Phase Transformer (Two Windings)1 : spsThreePhaseTransformerTwoWindingsLib/Three-Phase Transformer (Two Windings)  Winding1Connection=Yg  Winding2Connection=Yg  CoreType=Three single-phase transformers  SetSaturation=off  Hysteresis=off  DataFile='hysteresis'  SetInitialFlux=off  Measurements=None  UNITS=pu  NominalPower=[SG(1).TXR.Snom , Grid.f ]  Winding1=[ SG(1).Vbase , SG(1).TXR.R1 , SG(1).TXR.L1 ]  Winding2=[ Grid.Vbase , SG(1).TXR.R2 , SG(1).TXR.L2 ]  Rm=500  Lm=500  L0=2.866  Saturation=[ 0,0 ; 0.0024,1.2 ; 1.0,1.52 ]  InitialFluxes=[1273.5 -1273.5 1114.3]  BreakLoop=off  DiscreteSolver=Trapezoidal iterative  DataType=off  TransfoNumber=1
  Three-Phase Transformer (Two Windings)10 : spsThreePhaseTransformerTwoWindingsLib/Three-Phase Transformer (Two Windings)  Winding1Connection=Yg  Winding2Connection=Yg  CoreType=Three single-phase transformers  SetSaturation=off  Hysteresis=off  DataFile='hysteresis'  SetInitialFlux=off  Measurements=None  UNITS=pu  NominalPower=[IBR(2).TXR.Snom , Grid.f ]  Winding1=[ IBR(2).Vbase , IBR(2).TXR.R1 , IBR(2).TXR.L1 ]  Winding2=[ Grid.Vbase , IBR(2).TXR.R2 , IBR(2).TXR.L2 ]  Rm=600  Lm=500  L0=2.866  Saturation=[ 0,0 ; 0.0024,1.2 ; 1.0,1.52 ]  InitialFluxes=[1273.5 -1273.5 1114.3]  BreakLoop=off  DiscreteSolver=Trapezoidal iterative  DataType=off  TransfoNumber=1
  Three-Phase Transformer (Two Windings)2 : spsThreePhaseTransformerTwoWindingsLib/Three-Phase Transformer (Two Windings)  Winding1Connection=Yg  Winding2Connection=Yg  CoreType=Three single-phase transformers  SetSaturation=off  Hysteresis=off  DataFile='hysteresis'  SetInitialFlux=off  Measurements=None  UNITS=pu  NominalPower=[IBR(1).TXR.Snom , Grid.f ]  Winding1=[ IBR(1).Vbase , IBR(1).TXR.R1 , IBR(1).TXR.L1 ]  Winding2=[ Grid.Vbase , IBR(1).TXR.R2 , IBR(1).TXR.L2 ]  Rm=600  Lm=500  L0=2.866  Saturation=[ 0,0 ; 0.0024,1.2 ; 1.0,1.52 ]  InitialFluxes=[1273.5 -1273.5 1114.3]  BreakLoop=off  DiscreteSolver=Trapezoidal iterative  DataType=off  TransfoNumber=1
  Three-Phase Transformer (Two Windings)3 : spsThreePhaseTransformerTwoWindingsLib/Three-Phase Transformer (Two Windings)  Winding1Connection=Yg  Winding2Connection=Yg  CoreType=Three single-phase transformers  SetSaturation=off  Hysteresis=off  DataFile='hysteresis'  SetInitialFlux=off  Measurements=None  UNITS=pu  NominalPower=[SG(4).TXR.Snom , Grid.f ]  Winding1=[ SG(4).Vbase , SG(4).TXR.R1 , SG(4).TXR.L1 ]  Winding2=[ Grid.Vbase , SG(4).TXR.R2 , SG(4).TXR.L2 ]  Rm=500  Lm=500  L0=2.866  Saturation=[ 0,0 ; 0.0024,1.2 ; 1.0,1.52 ]  InitialFluxes=[1273.5 -1273.5 1114.3]  BreakLoop=off  DiscreteSolver=Trapezoidal iterative  DataType=off  TransfoNumber=1
  Three-Phase Transformer (Two Windings)4 : spsThreePhaseTransformerTwoWindingsLib/Three-Phase Transformer (Two Windings)  Winding1Connection=Yg  Winding2Connection=Yg  CoreType=Three single-phase transformers  SetSaturation=off  Hysteresis=off  DataFile='hysteresis'  SetInitialFlux=off  Measurements=None  UNITS=pu  NominalPower=[SG(5).TXR.Snom , Grid.f ]  Winding1=[ SG(5).Vbase , SG(5).TXR.R1 , SG(5).TXR.L1 ]  Winding2=[ Grid.Vbase , SG(5).TXR.R2 , SG(5).TXR.L2 ]  Rm=500  Lm=500  L0=2.866  Saturation=[ 0,0 ; 0.0024,1.2 ; 1.0,1.52 ]  InitialFluxes=[1273.5 -1273.5 1114.3]  BreakLoop=off  DiscreteSolver=Trapezoidal iterative  DataType=off  TransfoNumber=1
  Three-Phase Transformer (Two Windings)5 : spsThreePhaseTransformerTwoWindingsLib/Three-Phase Transformer (Two Windings)  Winding1Connection=Yg  Winding2Connection=Yg  CoreType=Three single-phase transformers  SetSaturation=off  Hysteresis=off  DataFile='hysteresis'  SetInitialFlux=off  Measurements=None  UNITS=pu  NominalPower=[IBR(2).TXR.Snom , Grid.f ]  Winding1=[ IBR(2).Vbase , IBR(2).TXR.R1 , IBR(2).TXR.L1 ]  Winding2=[ Grid.Vbase , IBR(2).TXR.R2 , IBR(2).TXR.L2 ]  Rm=600  Lm=500  L0=2.866  Saturation=[ 0,0 ; 0.0024,1.2 ; 1.0,1.52 ]  InitialFluxes=[1273.5 -1273.5 1114.3]  BreakLoop=off  DiscreteSolver=Trapezoidal iterative  DataType=off  TransfoNumber=1
  Three-Phase Transformer (Two Windings)6 : spsThreePhaseTransformerTwoWindingsLib/Three-Phase Transformer (Two Windings)  Winding1Connection=Yg  Winding2Connection=Yg  CoreType=Three single-phase transformers  SetSaturation=off  Hysteresis=off  DataFile='hysteresis'  SetInitialFlux=off  Measurements=None  UNITS=pu  NominalPower=[SG(2).TXR.Snom , Grid.f ]  Winding1=[ SG(2).Vbase , SG(2).TXR.R1 , SG(2).TXR.L1 ]  Winding2=[ Grid.Vbase , SG(2).TXR.R2 , SG(2).TXR.L2 ]  Rm=500  Lm=500  L0=2.866  Saturation=[ 0,0 ; 0.0024,1.2 ; 1.0,1.52 ]  InitialFluxes=[1273.5 -1273.5 1114.3]  BreakLoop=off  DiscreteSolver=Trapezoidal iterative  DataType=off  TransfoNumber=1
  Three-Phase Transformer (Two Windings)7 : spsThreePhaseTransformerTwoWindingsLib/Three-Phase Transformer (Two Windings)  Winding1Connection=Yg  Winding2Connection=Yg  CoreType=Three single-phase transformers  SetSaturation=off  Hysteresis=off  DataFile='hysteresis'  SetInitialFlux=off  Measurements=None  UNITS=pu  NominalPower=[SG(2).TXR.Snom , Grid.f ]  Winding1=[ SG(2).Vbase , SG(2).TXR.R1 , SG(2).TXR.L1 ]  Winding2=[ Grid.Vbase , SG(2).TXR.R2 , SG(2).TXR.L2 ]  Rm=500  Lm=500  L0=2.866  Saturation=[ 0,0 ; 0.0024,1.2 ; 1.0,1.52 ]  InitialFluxes=[1273.5 -1273.5 1114.3]  BreakLoop=off  DiscreteSolver=Trapezoidal iterative  DataType=off  TransfoNumber=1
  Three-Phase Transformer (Two Windings)8 : spsThreePhaseTransformerTwoWindingsLib/Three-Phase Transformer (Two Windings)  Winding1Connection=Yg  Winding2Connection=Yg  CoreType=Three single-phase transformers  SetSaturation=off  Hysteresis=off  DataFile='hysteresis'  SetInitialFlux=off  Measurements=None  UNITS=pu  NominalPower=[IBR(3).TXR.Snom , Grid.f ]  Winding1=[ IBR(3).Vbase , IBR(3).TXR.R1 , IBR(3).TXR.L1 ]  Winding2=[ Grid.Vbase , IBR(3).TXR.R2 , IBR(3).TXR.L2 ]  Rm=500  Lm=500  L0=2.866  Saturation=[ 0,0 ; 0.0024,1.2 ; 1.0,1.52 ]  InitialFluxes=[1273.5 -1273.5 1114.3]  BreakLoop=off  DiscreteSolver=Trapezoidal iterative  DataType=off  TransfoNumber=1
  Three-Phase Transformer (Two Windings)9 : spsThreePhaseTransformerTwoWindingsLib/Three-Phase Transformer (Two Windings)  Winding1Connection=Yg  Winding2Connection=Yg  CoreType=Three single-phase transformers  SetSaturation=off  Hysteresis=off  DataFile='hysteresis'  SetInitialFlux=off  Measurements=None  UNITS=pu  NominalPower=[SG(6).TXR.Snom , Grid.f ]  Winding1=[ SG(6).Vbase , SG(6).TXR.R1 , SG(6).TXR.L1 ]  Winding2=[ Grid.Vbase , SG(6).TXR.R2 , SG(6).TXR.L2 ]  Rm=500  Lm=500  L0=2.866  Saturation=[ 0,0 ; 0.0024,1.2 ; 1.0,1.52 ]  InitialFluxes=[1273.5 -1273.5 1114.3]  BreakLoop=off  DiscreteSolver=Trapezoidal iterative  DataType=off  TransfoNumber=1
  Three-Phase Breaker : spsThreePhaseBreakerLib/Three-Phase Breaker  InitialState=open  SwitchA=on  SwitchB=on  SwitchC=on  SwitchTimes=[13]  External=off  BreakerResistance=0.01  SnubberResistance=1e6  SnubberCapacitance=inf  Measurements=None
  Three-Phase Breaker1 : spsThreePhaseBreakerLib/Three-Phase Breaker  InitialState=open  SwitchA=on  SwitchB=on  SwitchC=on  SwitchTimes=[13 23]  External=off  BreakerResistance=0.01  SnubberResistance=1e6  SnubberCapacitance=inf  Measurements=None
  Three-Phase Breaker2 : spsThreePhaseBreakerLib/Three-Phase Breaker  InitialState=open  SwitchA=on  SwitchB=on  SwitchC=on  SwitchTimes=[40]  External=off  BreakerResistance=0.01  SnubberResistance=1e6  SnubberCapacitance=inf  Measurements=None
  To Workspace1 : ToWorkspace  VariableName=SG5_u  SaveFormat=Timeseries  SampleTime=10^(-4)
  To Workspace10 : ToWorkspace  VariableName=SG5_omega  SaveFormat=Timeseries  SampleTime=10^(-4)
  To Workspace11 : ToWorkspace  VariableName=delta1  SaveFormat=Timeseries  SampleTime=10^(-4)
  To Workspace12 : ToWorkspace  VariableName=SG6_omega  SaveFormat=Timeseries  SampleTime=10^(-4)
  To Workspace13 : ToWorkspace  VariableName=delta2  SaveFormat=Timeseries  SampleTime=10^(-4)
  To Workspace14 : ToWorkspace  VariableName=delta3  SaveFormat=Timeseries  SampleTime=10^(-4)
  To Workspace15 : ToWorkspace  VariableName=delta4  SaveFormat=Timeseries  SampleTime=10^(-4)
  To Workspace16 : ToWorkspace  VariableName=delta5  SaveFormat=Timeseries  SampleTime=10^(-4)
  To Workspace17 : ToWorkspace  VariableName=delta6  SaveFormat=Timeseries  SampleTime=10^(-4)
  To Workspace18 : ToWorkspace  VariableName=x_IBR1  SaveFormat=Timeseries  SampleTime=10^(-4)
  To Workspace19 : ToWorkspace  VariableName=x_IBR2  SaveFormat=Timeseries  SampleTime=10^(-4)
  To Workspace2 : ToWorkspace  VariableName=SG1_u  SaveFormat=Timeseries  SampleTime=10^(-4)
  To Workspace20 : ToWorkspace  VariableName=x_IBR3  SaveFormat=Timeseries  SampleTime=10^(-4)
  To Workspace21 : ToWorkspace  VariableName=SG4_f  SaveFormat=Timeseries  SampleTime=10^(-4)
  To Workspace22 : ToWorkspace  VariableName=SG5_f  SaveFormat=Timeseries  SampleTime=10^(-4)
  To Workspace23 : ToWorkspace  VariableName=SG6_f  SaveFormat=Timeseries  SampleTime=10^(-4)
  To Workspace24 : ToWorkspace  VariableName=SG3_u  SaveFormat=Timeseries  SampleTime=10^(-4)
  To Workspace25 : ToWorkspace  VariableName=SG1_p  SaveFormat=Timeseries  SampleTime=10^(-4)
  To Workspace26 : ToWorkspace  VariableName=SG2_p  SaveFormat=Timeseries  SampleTime=10^(-4)
  To Workspace27 : ToWorkspace  VariableName=SG3_p  SaveFormat=Timeseries  SampleTime=10^(-4)
  To Workspace28 : ToWorkspace  VariableName=SG4_p  SaveFormat=Timeseries  SampleTime=10^(-4)
  To Workspace29 : ToWorkspace  VariableName=SG5_p  SaveFormat=Timeseries  SampleTime=10^(-4)
  To Workspace3 : ToWorkspace  VariableName=SG1_f  SaveFormat=Timeseries  SampleTime=10^(-4)
  To Workspace30 : ToWorkspace  VariableName=SG6_p  SaveFormat=Timeseries  SampleTime=10^(-4)
  To Workspace31 : ToWorkspace  VariableName=IBR1_p  SaveFormat=Timeseries  SampleTime=10^(-4)
  To Workspace32 : ToWorkspace  VariableName=IBR2_p  SaveFormat=Timeseries  SampleTime=10^(-4)
  To Workspace33 : ToWorkspace  VariableName=IBR3_p  SaveFormat=Timeseries  SampleTime=10^(-4)
  To Workspace34 : ToWorkspace  VariableName=load  SaveFormat=Timeseries  SampleTime=10^(-4)
  To Workspace35 : ToWorkspace  VariableName=x_IBR4  SaveFormat=Timeseries  SampleTime=10^(-4)
  To Workspace36 : ToWorkspace  VariableName=IBR4_p  SaveFormat=Timeseries  SampleTime=10^(-4)
  To Workspace4 : ToWorkspace  VariableName=SG2_f  SaveFormat=Timeseries  SampleTime=10^(-4)
  To Workspace5 : ToWorkspace  VariableName=SG3_f  SaveFormat=Timeseries  SampleTime=10^(-4)
  To Workspace6 : ToWorkspace  VariableName=SG1_omega  SaveFormat=Timeseries  SampleTime=10^(-4)
  To Workspace7 : ToWorkspace  VariableName=SG2_omega  SaveFormat=Timeseries  SampleTime=10^(-4)
  To Workspace8 : ToWorkspace  VariableName=SG3_omega  SaveFormat=Timeseries  SampleTime=10^(-4)
  To Workspace9 : ToWorkspace  VariableName=SG4_omega  SaveFormat=Timeseries  SampleTime=10^(-4)
  powergui : sps_lib/powergui  Priority=1  SimulationMode=Discrete  SampleTime=Ts  frequency=60  Iterations=50  frequencyindice=0  Pbase=100e6  ErrMax=1e-4  UnitsV=kV  UnitsW=MW  buscounter=0  FunctionMessages=off  echomessages=off  EnableUseOfTLC=off  CurrentSourceSwitches=off  DisableSnubberDevices=off  DisableRonSwitches=off  DisableVfSwitches=off  DisplayEquations=off  AutomaticDiscreteSolvers=off  SolverType=Tustin/Backward Euler (TBE)  Interpol=off  ExternalGateDelay=off  methode=off  Ts=100  x0status=blocks  SPID=on  SwTol=0  HookPort=off  NonlinearTolerance=1e-4  nMaxIteration=100  ContinueOnMaxIteration=off  RestoreLinks=warning  ResistiveCurrentMeasurement=off  Frange=[0:2:500]  Ylog=off  Xlog=on  ShowGrid=off  save=off  variable=ZData  structure=0  ZoomFFT=off  StartTime=0.0  cycles=1  DisplayStyle=1  fundamental=60  FreqAxis=off  MaxFrequency=1000  frequencyindicesteady=1  RmsSteady=1  display=off
  wires:
  Bus Selector23/2 -> Display8/1  "<Q>"
  Bus Selector23/1 -> Display7/1  "<P>"
  [B8_IBR2] -> IBR2/3(Inport)
  [B8_IBR2] -> Bus Selector23/1
  [B8_wt] -> IBR2/4(Inport1)
  IBR2/1(Outport) -> [m_IBR2]
  Constant2/1 -> IBR2/1(In1)
  PLL (3ph)/2(wt) -> [B8_wt]
  PLL (3ph)/1(Freq) -> Display6/1
  [B1_SG1] -> Bus Selector1/1
  Bus Selector1/1 -> Display1/1  "<P>"
  Bus Selector1/2 -> Display2/1  "<Q>"
  Bus Selector2/1 -> Display3/1  "<P>"
  Bus Selector2/2 -> Display4/1  "<Q>"
  [B9_L] -> Bus Selector2/1
  [m_SG1] -> Bus Selector3/1
  Bus Selector3/1 -> Display5/1  "<Rotor speed wm (pu)>"
  [m_SG1] -> Bus Selector7/1
  Bus Selector7/1 -> Gain1/1  "<Rotor speed wm (pu)>"
  [B1_SG1] -> Bus Selector10/1
  [B8_SG3] -> Bus Selector15/1
  Bus Selector15/1 -> PLL (3ph)/1(abc)  "<V>"
  [B1_IBR1] -> Bus Selector19/1
  Bus Selector1/3 -> Display9/1  "<Vmag>"
  Bus Selector1/4 -> Display10/1  "<Vphase>"
  Constant1/1 -> Add/1
  Bus Selector26/2 -> Display13/1  "<Q>"
  Bus Selector26/1 -> Display12/1  "<P>"
  [B1_IBR1] -> Bus Selector26/1
  Gain1/1 -> To Workspace3/1, Scope/1
  Gain10/1 -> To Workspace4/1, Scope/2
  Bus Selector30/1 -> Gain10/1  "<Rotor speed wm (pu)>"
  [m_SG2] -> Bus Selector30/1
  [B8_IBR2] -> Bus Selector32/1
  Gain2/1 -> Add/3
  [m_SG1] -> Bus Selector4/1
  Bus Selector4/1 -> Gain2/1  "<Rotor speed wm (pu)>"
  Constant14/1 -> Gain3/1
  Gain3/1 -> Add/2
  Add/1 -> SG1/1
  Constant/1 -> SG1/2
  Gain17/1 -> Add6/3
  Gain18/1 -> Add6/2
  [m_SG2] -> Bus Selector9/1
  Constant19/1 -> Gain18/1
  Bus Selector9/1 -> Gain17/1  "<Rotor speed wm (pu)>"
  Constant21/1 -> Add6/1
  Add6/1 -> SG2/1
  Constant20/1 -> SG2/2
  SG2/1 -> [m_SG2]
  Gain19/1 -> Add7/3
  SG3/1 -> [m_SG3]
  Add7/1 -> SG3/1
  Constant22/1 -> Gain20/1
  Constant24/1 -> SG3/2
  Bus Selector12/1 -> Gain19/1  "<Rotor speed wm (pu)>"
  [m_SG3] -> Bus Selector12/1
  Constant25/1 -> Add7/1
  Gain20/1 -> Add7/2
  SG1/1 -> [m_SG1]
  IBR1/1(Outport) -> [m_IBR1]
  [B1_IBR1] -> IBR1/3(Inport)
  [B1_wt] -> IBR1/4(Inport1)
  [m_SG3] -> Bus Selector5/1
  Bus Selector5/1 -> Gain11/1  "<Rotor speed wm (pu)>"
  Gain11/1 -> To Workspace5/1, Scope/3
  [B9_SG2] -> Bus Selector8/1
  [B8_SG3] -> Bus Selector11/1
  PLL (3ph)1/1(Freq) -> Display11/1
  PLL (3ph)1/2(wt) -> [B1_wt]
  Bus Selector14/1 -> PLL (3ph)1/1(abc)  "<V>"
  [B1_SG1] -> Bus Selector14/1
  SG4/1 -> [m_SG4]
  Bus Selector22/1 -> Gain12/1  "<Rotor speed wm (pu)>"
  Constant15/1 -> Add20/1
  Gain21/1 -> Add20/2
  Constant12/1 -> Gain21/1
  Gain12/1 -> Add20/3
  [m_SG4] -> Bus Selector22/1
  Add20/1 -> SG4/1
  Constant17/1 -> SG4/2
  Bus Selector27/1 -> Display14/1  "<P>"
  [B7_L] -> Bus Selector27/1
  Bus Selector27/2 -> Display15/1  "<Q>"
  Bus Selector29/2 -> Display18/1  "<Q>"
  Bus Selector29/4 -> Display17/1  "<Vphase>"
  [B8_SG3] -> Bus Selector29/1
  Bus Selector29/3 -> Display19/1  "<Vmag>"
  Bus Selector29/1 -> Display16/1  "<P>"
  Bus Selector31/1 -> Display20/1  "<P>"
  Bus Selector31/3 -> Display23/1  "<Vmag>"
  Bus Selector31/4 -> Display21/1  "<Vphase>"
  [B9_SG2] -> Bus Selector31/1
  Bus Selector31/2 -> Display22/1  "<Q>"
  Bus Selector33/1 -> Display24/1  "<P>"
  Bus Selector33/3 -> Display27/1  "<Vmag>"
  Bus Selector33/4 -> Display25/1  "<Vphase>"
  [B7_SG4] -> Bus Selector33/1
  Bus Selector33/2 -> Display26/1  "<Q>"
  Constant18/1 -> Gain23/1
  Gain23/1 -> Add21/2
  Constant26/1 -> Add21/1
  Bus Selector34/1 -> Gain22/1  "<Rotor speed wm (pu)>"
  Gain22/1 -> Add21/3
  [m_SG5] -> Bus Selector34/1
  SG5/1 -> [m_SG5]
  Constant23/1 -> SG5/2
  Add21/1 -> SG5/1
  [B6_IBR3] -> IBR3/3(Inport)
  Bus Selector36/2 -> Display30/1  "<Q>"
  [B6_IBR3] -> Bus Selector36/1
  IBR3/1(Outport) -> [m_IBR3]
  [B6_wt] -> IBR3/4(Inport1)
  PLL (3ph)2/2(wt) -> [B6_wt]
  PLL (3ph)2/1(Freq) -> Display28/1
  [B6_SG5] -> Bus Selector35/1
  Bus Selector36/1 -> Display29/1  "<P>"
  [m_SG6] -> Bus Selector37/1
  Constant27/1 -> Gain25/1
  Constant28/1 -> SG6/2
  Gain25/1 -> Add22/2
  Bus Selector37/1 -> Gain24/1  "<Rotor speed wm (pu)>"
  Add22/1 -> SG6/1
  Gain24/1 -> Add22/3
  Constant29/1 -> Add22/1
  SG6/1 -> [m_SG6]
  Bus Selector38/1 -> Display31/1  "<P>"
  [B5_L] -> Bus Selector38/1
  Bus Selector38/2 -> Display32/1  "<Q>"
  Bus Selector39/1 -> Gain26/1  "<Rotor speed wm (pu)>"
  [m_SG4] -> Bus Selector39/1
  Gain26/1 -> To Workspace21/1, Scope/4
  Bus Selector40/1 -> Gain27/1  "<Rotor speed wm (pu)>"
  Gain27/1 -> To Workspace22/1, Scope/5
  [m_SG5] -> Bus Selector40/1
  Gain28/1 -> To Workspace23/1, Scope/6
  Bus Selector41/1 -> Gain28/1  "<Rotor speed wm (pu)>"
  [m_SG6] -> Bus Selector41/1
  [B6_SG5] -> Bus Selector42/1
  Bus Selector10/1 -> Scope1/1, To Workspace25/1  "<P>"
  Bus Selector8/1 -> To Workspace26/1, Scope1/2  "<P>"
  Bus Selector11/1 -> To Workspace27/1, Scope1/3  "<P>"
  Bus Selector42/1 -> To Workspace29/1, Scope1/5  "<P>"
  Bus Selector43/1 -> To Workspace30/1, Scope1/6  "<P>"
  [B5_SG6] -> Bus Selector43/1
  Bus Selector44/1 -> To Workspace28/1, Scope1/4  "<P>"
  [B7_SG4] -> Bus Selector44/1
  Bus Selector19/1 -> To Workspace31/1, Scope2/1  "<P>"
  Bus Selector32/1 -> To Workspace32/1, Scope2/2  "<P>"
  Bus Selector45/1 -> To Workspace33/1, Scope2/3  "<P>"
  [B6_IBR3] -> Bus Selector45/1
  [m_SG2] -> Bus Selector54/1
  Bus Selector54/1 -> Display33/1  "<Rotor speed wm (pu)>"
  Bus Selector35/1 -> PLL (3ph)2/1(abc)  "<V>"
  Bus Selector91/3 -> Display37/1  "<Vmag>"
  Bus Selector91/4 -> Display35/1  "<Vphase>"
  Bus Selector91/1 -> Display34/1  "<P>"
  Bus Selector91/2 -> Display36/1  "<Q>"
  [B6_SG5] -> Bus Selector91/1
  Bus Selector92/3 -> Display41/1  "<Vmag>"
  Bus Selector92/4 -> Display39/1  "<Vphase>"
  Bus Selector92/1 -> Display38/1  "<P>"
  Bus Selector92/2 -> Display40/1  "<Q>"
  [B5_SG6] -> Bus Selector92/1
  Constant3/1 -> IBR3/1(In1)
  Constant4/1 -> IBR1/1(In1)
  Constant5/1 -> Sum/1
  Sum/1 -> Integrator/1
  Integrator/1 -> Gain4/1
  Constant6/1 -> Sum1/1
  Sum1/1 -> Integrator1/1
  Integrator1/1 -> Gain5/1
  Bus Selector6/1 -> Sum1/2  "<Rotor speed wm (pu)>"
  [m_SG3] -> Bus Selector6/1
  [m_SG1] -> Bus Selector13/1
  Bus Selector13/1 -> Sum/2  "<Rotor speed wm (pu)>"
  Clock/1 -> Switch/2
  Gain5/1 -> Switch/1
  Switch/1 -> To Workspace24/1, Add7/4
  Switch1/1 -> To Workspace2/1, Add/4
  Gain4/1 -> Switch1/1
  Clock1/1 -> Switch1/2
  [m_SG5] -> Bus Selector16/1
  Bus Selector16/1 -> Sum2/2  "<Rotor speed wm (pu)>"
  Gain6/1 -> Switch2/1
  Switch2/1 -> To Workspace1/1, Add21/4
  Integrator2/1 -> Gain6/1
  Clock2/1 -> Switch2/2
  Constant7/1 -> Sum2/1
  Sum2/1 -> Integrator2/1
  Bus Selector51/1 -> Add17/2  "<Rotor speed wm (pu)>"
  [m_SG6] -> Bus Selector53/1
  Add11/1 -> To Workspace7/1
  Bus Selector52/1 -> Add36/2  "<Rotor speed wm (pu)>"
  Bus Selector18/1 -> Add18/2  "<Rotor speed wm (pu)>"
  [m_SG1] -> Bus Selector21/1
  Constant38/1 -> Add35/1
  Add9/1 -> To Workspace6/1
  [m_SG2] -> Bus Selector24/1
  Bus Selector50/1 -> Add35/2  "<Rotor speed wm (pu)>"
  Add13/1 -> To Workspace8/1
  Integrator14/1 -> To Workspace17/1
  Add18/1 -> Integrator12/1
  [m_SG3] -> Bus Selector51/1
  Integrator3/1 -> To Workspace11/1
  Integrator4/1 -> To Workspace13/1
  Constant40/1 -> Add36/1
  Bus Selector25/1 -> Add9/2  "<Rotor speed wm (pu)>"
  [m_SG4] -> Bus Selector17/1
  Add34/1 -> To Workspace10/1
  Constant9/1 -> Add12/1
  Add36/1 -> Integrator13/1
  [m_SG4] -> Bus Selector18/1
  Constant16/1 -> Add13/1
  Bus Selector21/1 -> Add38/2  "<Rotor speed wm (pu)>"
  Add17/1 -> Integrator5/1
  [m_IBR3] -> To Workspace20/1
  [m_SG2] -> Bus Selector20/1
  Bus Selector17/1 -> Add33/2  "<Rotor speed wm (pu)>"
  Bus Selector24/1 -> Add11/2  "<Rotor speed wm (pu)>"
  Constant11/1 -> Add17/1
  Constant10/1 -> Add9/1
  Constant8/1 -> Add38/1
  [m_SG1] -> Bus Selector25/1
  Constant37/1 -> Add34/1
  Bus Selector28/1 -> Add13/2  "<Rotor speed wm (pu)>"
  [m_IBR2] -> To Workspace19/1
  Add38/1 -> Integrator3/1
  [m_SG5] -> Bus Selector52/1
  Add37/1 -> Integrator14/1
  [m_SG5] -> Bus Selector49/1
  Constant13/1 -> Add11/1
  Bus Selector49/1 -> Add34/2  "<Rotor speed wm (pu)>"
  Constant41/1 -> Add37/1
  [m_SG3] -> Bus Selector28/1
  [m_IBR1] -> To Workspace18/1
  Add12/1 -> Integrator4/1
  Integrator12/1 -> To Workspace15/1
  Constant39/1 -> Add18/1
  Add35/1 -> To Workspace12/1
  [m_SG6] -> Bus Selector50/1
  Integrator13/1 -> To Workspace16/1
  Bus Selector53/1 -> Add37/2  "<Rotor speed wm (pu)>"
  Bus Selector20/1 -> Add12/2  "<Rotor speed wm (pu)>"
  Constant36/1 -> Add33/1
  Add33/1 -> To Workspace9/1
  Integrator5/1 -> To Workspace14/1
  [B1_IBR1] -> Bus Selector46/1
  Bus Selector46/1 -> ?  "<P>"
  [B9_L] -> Bus Selector47/1
  [B5_L] -> Bus Selector48/1
  [B7_L] -> Bus Selector55/1
  Bus Selector47/1 -> Add1/1  "<P>"
  Bus Selector48/1 -> Add1/2  "<P>"
  Bus Selector55/1 -> Add1/3  "<P>"
  Add1/1 -> To Workspace34/1, Scope3/1
  PLL (3ph)3/1(Freq) -> Display42/1
  [B7_SG4] -> Bus Selector56/1
  [B7_IBR4] -> IBR4/3(Inport)
  [B7_IBR4] -> Bus Selector57/1
  Bus Selector57/2 -> Display44/1  "<Q>"
  IBR4/1(Outport) -> [m_IBR4]
  PLL (3ph)3/2(wt) -> [B7_wt]
  [B7_wt] -> IBR4/4(Inport1)
  Constant30/1 -> IBR4/1(In1)
  Bus Selector57/1 -> Display43/1  "<P>"
  Bus Selector56/1 -> PLL (3ph)3/1(abc)  "<V>"
  [m_IBR4] -> To Workspace35/1
  Bus Selector58/1 -> Scope2/4, To Workspace36/1  "<P>"
  [B7_IBR4] -> Bus Selector58/1
  connections:
  Three-Phase Series RLC Load2/LConn1 -- SG1/RConn1 -- Three-Phase Transformer (Two Windings)1/LConn1
  Three-Phase Series RLC Load2/LConn2 -- SG1/RConn2 -- Three-Phase Transformer (Two Windings)1/LConn2
  Three-Phase Series RLC Load2/LConn3 -- SG1/RConn3 -- Three-Phase Transformer (Two Windings)1/LConn3
  IBR2/RConn3 -- Three-Phase Transformer (Two Windings)5/LConn3
  B8_IBR2/LConn2 -- Three-Phase Transformer (Two Windings)5/RConn2
  B8_IBR2/LConn3 -- Three-Phase Transformer (Two Windings)5/RConn3
  B8_IBR2/LConn1 -- Three-Phase Transformer (Two Windings)5/RConn1
  IBR2/RConn2 -- Three-Phase Transformer (Two Windings)5/LConn2
  Ground4/LConn1 -- IBR2/LConn1
  IBR2/RConn1 -- Three-Phase Transformer (Two Windings)5/LConn1
  Three-Phase Transformer (Two Windings)1/RConn1 -- B1_SG1/LConn1
  Three-Phase Transformer (Two Windings)1/RConn2 -- B1_SG1/LConn2
  Three-Phase Transformer (Two Windings)1/RConn3 -- B1_SG1/LConn3
  Three-Phase Series RLC Load1/LConn1 -- Three-Phase Breaker/LConn1
  Three-Phase Series RLC Load1/LConn2 -- Three-Phase Breaker/LConn2
  Three-Phase Series RLC Load1/LConn3 -- Three-Phase Breaker/LConn3
  Three-Phase Transformer (Two Windings)6/LConn1 -- SG2/RConn1 -- Three-Phase Series RLC Load4/LConn1
  Three-Phase Series RLC Load4/LConn2 -- SG2/RConn2 -- Three-Phase Transformer (Two Windings)6/LConn2
  Three-Phase Series RLC Load4/LConn3 -- SG2/RConn3 -- Three-Phase Transformer (Two Windings)6/LConn3
  B9_SG2/LConn1 -- Three-Phase Transformer (Two Windings)6/RConn1
  B9_SG2/LConn2 -- Three-Phase Transformer (Two Windings)6/RConn2
  B9_SG2/LConn3 -- Three-Phase Transformer (Two Windings)6/RConn3
  B9_SG2/RConn1 -- B9_L/LConn1 -- TX1/LConn1 -- TX2/RConn1
  B9_SG2/RConn2 -- B9_L/LConn2 -- TX2/RConn2 -- TX1/LConn2
  B9_SG2/RConn3 -- B9_L/LConn3 -- TX1/LConn3 -- TX2/RConn3
  Three-Phase Series RLC Load5/LConn3 -- SG3/RConn3 -- Three-Phase Transformer (Two Windings)7/LConn3
  Three-Phase Series RLC Load5/LConn2 -- SG3/RConn2 -- Three-Phase Transformer (Two Windings)7/LConn2
  Three-Phase Transformer (Two Windings)7/LConn1 -- SG3/RConn1 -- Three-Phase Series RLC Load5/LConn1
  B8_SG3/LConn1 -- Three-Phase Transformer (Two Windings)7/RConn1
  B8_SG3/LConn3 -- Three-Phase Transformer (Two Windings)7/RConn3
  B8_SG3/LConn2 -- Three-Phase Transformer (Two Windings)7/RConn2
  Three-Phase Transformer (Two Windings)2/LConn1 -- IBR1/RConn1
  Three-Phase Transformer (Two Windings)2/LConn2 -- IBR1/RConn2
  IBR1/RConn3 -- Three-Phase Transformer (Two Windings)2/LConn3
  Three-Phase Transformer (Two Windings)2/RConn1 -- B1_IBR1/LConn1
  Three-Phase Transformer (Two Windings)2/RConn2 -- B1_IBR1/LConn2
  Three-Phase Transformer (Two Windings)2/RConn3 -- B1_IBR1/LConn3
  Ground1/LConn1 -- IBR1/LConn1
  B7_SG4/LConn1 -- Three-Phase Transformer (Two Windings)3/RConn1
  B7_SG4/LConn3 -- Three-Phase Transformer (Two Windings)3/RConn3
  B7_SG4/LConn2 -- Three-Phase Transformer (Two Windings)3/RConn2
  TX3/RConn1 -- TX4/LConn1 -- B7_IBR4/RConn1 -- B7_L/LConn1 -- B7_SG4/RConn1
  TX3/RConn2 -- TX4/LConn2 -- B7_IBR4/RConn2 -- B7_L/LConn2 -- B7_SG4/RConn2
  TX3/RConn3 -- B7_IBR4/RConn3 -- B7_L/LConn3 -- B7_SG4/RConn3 -- TX4/LConn3
  SG4/RConn1 -- Three-Phase Series RLC Load11/LConn1 -- Three-Phase Transformer (Two Windings)3/LConn1
  SG4/RConn2 -- Three-Phase Series RLC Load11/LConn2 -- Three-Phase Transformer (Two Windings)3/LConn2
  SG4/RConn3 -- Three-Phase Series RLC Load11/LConn3 -- Three-Phase Transformer (Two Windings)3/LConn3
  Three-Phase Series RLC Load3/LConn1 -- Three-Phase Breaker1/RConn1 -- B7_L/RConn1
  Three-Phase Series RLC Load3/LConn3 -- Three-Phase Breaker1/RConn3 -- B7_L/RConn3
  Three-Phase Series RLC Load3/LConn2 -- B7_L/RConn2 -- Three-Phase Breaker1/RConn2
  Three-Phase Series RLC Load6/LConn3 -- Three-Phase Breaker1/LConn3
  Three-Phase Series RLC Load6/LConn2 -- Three-Phase Breaker1/LConn2
  Three-Phase Series RLC Load6/LConn1 -- Three-Phase Breaker1/LConn1
  TX4/RConn2 -- Three-Phase Parallel RLC Load1/LConn2 -- B6_IBR3/RConn2 -- TX5/RConn2 -- B6_SG5/RConn2
  B6_SG5/LConn1 -- Three-Phase Transformer (Two Windings)4/RConn1
  B6_SG5/LConn2 -- Three-Phase Transformer (Two Windings)4/RConn2
  B6_SG5/LConn3 -- Three-Phase Transformer (Two Windings)4/RConn3
  SG5/RConn1 -- Three-Phase Series RLC Load7/LConn1 -- Three-Phase Transformer (Two Windings)4/LConn1
  SG5/RConn2 -- Three-Phase Series RLC Load7/LConn2 -- Three-Phase Transformer (Two Windings)4/LConn2
  SG5/RConn3 -- Three-Phase Series RLC Load7/LConn3 -- Three-Phase Transformer (Two Windings)4/LConn3
  Ground2/LConn1 -- IBR3/LConn1
  Three-Phase Transformer (Two Windings)8/LConn1 -- IBR3/RConn1
  Three-Phase Transformer (Two Windings)8/LConn2 -- IBR3/RConn2
  Three-Phase Transformer (Two Windings)8/LConn3 -- IBR3/RConn3
  Three-Phase Series RLC Load8/LConn2 -- SG6/RConn2 -- Three-Phase Transformer (Two Windings)9/LConn2
  Three-Phase Series RLC Load8/LConn1 -- SG6/RConn1 -- Three-Phase Transformer (Two Windings)9/LConn1
  Three-Phase Series RLC Load8/LConn3 -- SG6/RConn3 -- Three-Phase Transformer (Two Windings)9/LConn3
  B5_SG6/LConn2 -- Three-Phase Transformer (Two Windings)9/RConn2
  B5_SG6/LConn1 -- Three-Phase Transformer (Two Windings)9/RConn1
  B5_SG6/LConn3 -- Three-Phase Transformer (Two Windings)9/RConn3
  B5_L/LConn1 -- TX6/RConn1 -- TX5/LConn1 -- B5_SG6/RConn1
  TX6/RConn2 -- TX5/LConn2 -- B5_L/LConn2 -- B5_SG6/RConn2
  B5_L/LConn3 -- TX6/RConn3 -- TX5/LConn3 -- B5_SG6/RConn3
  Three-Phase Series RLC Load10/LConn2 -- Three-Phase Breaker2/LConn2
  Three-Phase Series RLC Load10/LConn3 -- Three-Phase Breaker2/LConn3
  Three-Phase Series RLC Load10/LConn1 -- Three-Phase Breaker2/LConn1
  TX4/RConn1 -- Three-Phase Parallel RLC Load1/LConn1 -- B6_IBR3/RConn1 -- TX5/RConn1 -- B6_SG5/RConn1
  TX4/RConn3 -- TX5/RConn3 -- Three-Phase Parallel RLC Load1/LConn3 -- B6_IBR3/RConn3 -- B6_SG5/RConn3
  B8_SG3/RConn1 -- B8_IBR2/RConn1 -- TX3/LConn1 -- TX2/LConn1
  B8_SG3/RConn2 -- B8_IBR2/RConn2 -- TX3/LConn2 -- TX2/LConn2
  B8_SG3/RConn3 -- B8_IBR2/RConn3 -- TX3/LConn3 -- TX2/LConn3
  B6_IBR3/LConn1 -- Three-Phase Transformer (Two Windings)8/RConn1
  B6_IBR3/LConn2 -- Three-Phase Transformer (Two Windings)8/RConn2
  B6_IBR3/LConn3 -- Three-Phase Transformer (Two Windings)8/RConn3
  TX1/RConn1 -- TX6/LConn1 -- B1_IBR1/RConn1 -- B1_SG1/RConn1
  TX1/RConn2 -- TX6/LConn2 -- B1_IBR1/RConn2 -- B1_SG1/RConn2
  TX1/RConn3 -- TX6/LConn3 -- B1_IBR1/RConn3 -- B1_SG1/RConn3
  Three-Phase Parallel RLC Load/LConn1 -- Three-Phase Breaker2/RConn1 -- B5_L/RConn1
  B5_L/RConn2 -- Three-Phase Breaker2/RConn2 -- Three-Phase Parallel RLC Load/LConn2
  Three-Phase Parallel RLC Load/LConn3 -- Three-Phase Breaker2/RConn3 -- B5_L/RConn3
  Three-Phase Parallel RLC Load2/LConn1 -- Three-Phase Breaker/RConn1 -- B9_L/RConn1
  Three-Phase Parallel RLC Load2/LConn2 -- B9_L/RConn2 -- Three-Phase Breaker/RConn2
  Three-Phase Parallel RLC Load2/LConn3 -- Three-Phase Breaker/RConn3 -- B9_L/RConn3
  IBR4/RConn3 -- Three-Phase Transformer (Two Windings)10/LConn3
  B7_IBR4/LConn2 -- Three-Phase Transformer (Two Windings)10/RConn2
  B7_IBR4/LConn3 -- Three-Phase Transformer (Two Windings)10/RConn3
  Ground3/LConn1 -- IBR4/LConn1
  B7_IBR4/LConn1 -- Three-Phase Transformer (Two Windings)10/RConn1
  IBR4/RConn2 -- Three-Phase Transformer (Two Windings)10/LConn2
  IBR4/RConn1 -- Three-Phase Transformer (Two Windings)10/LConn1
